simulink library "vehicle_model"  (R2018b)
settings: Solver=ode45  StartTime=0.0  StopTime=10.0  RelTol=1e-3  EnableMultiTasking=on
undefined symbols (not defined in the file): DiscIntNeverNeededParam, par_VEH, select_To_Wks_akt, stepsize, v0
libraries: $bdroot x8, pacejka_trans x6, simulink x4, body_chassis_vert x1
(part 2 of 4)

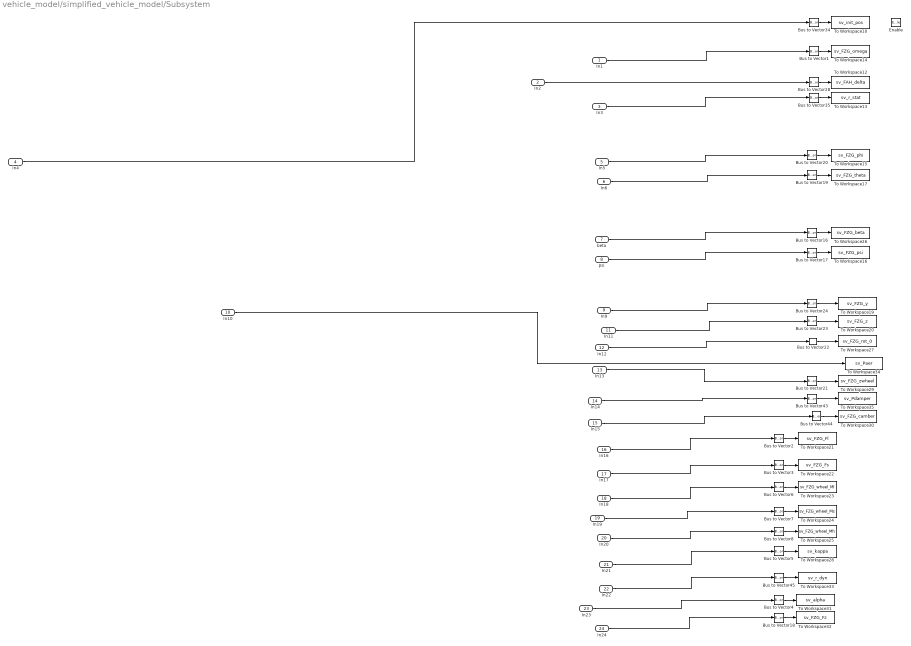
== system vehicle_model/simplified_vehicle_model/Subsystem ==
  In1 : Inport
  In2 : Inport  Port=2
  In3 : Inport  Port=3
  In4 : Inport  Port=4
  In5 : Inport  Port=5
  In6 : Inport  Port=6
  beta : Inport  Port=7
  psi : Inport  Port=8
  In9 : Inport  Port=9
  In10 : Inport  Port=10
  In11 : Inport  Port=11
  In12 : Inport  Port=12
  In13 : Inport  Port=13
  In14 : Inport  Port=14
  In15 : Inport  Port=15
  In16 : Inport  Port=16
  In17 : Inport  Port=17
  In18 : Inport  Port=18
  In19 : Inport  Port=19
  In20 : Inport  Port=20
  In21 : Inport  Port=21
  In22 : Inport  Port=22
  In23 : Inport  Port=23
  In24 : Inport  Port=24
  Enable : EnablePort
  Bus to Vector{1..8,16..24,28,34..35,43..45} (23 alike) : BusToVector
  To Workspace10 : ToWorkspace  VariableName=sv_init_pos  SampleTime=-1
      settings: MaxDataPoints=1  Decimation=savedec  Save2DSignal=2-D array (concatenate along first dimension)
  To Workspace12 : ToWorkspace  VariableName=sv_FAH_delta  SampleTime=-1
      settings: Decimation=savedec  Save2DSignal=2-D array (concatenate along first dimension)
  To Workspace13 : ToWorkspace  VariableName=sv_r_stat  SampleTime=-1
      settings: Decimation=savedec  Save2DSignal=2-D array (concatenate along first dimension)
  To Workspace14 : ToWorkspace  VariableName=sv_FZG_omega  SampleTime=-1
      settings: Decimation=savedec  Save2DSignal=2-D array (concatenate along first dimension)
  To Workspace15 : ToWorkspace  VariableName=sv_FZG_phi  SampleTime=-1
      settings: Decimation=savedec  Save2DSignal=2-D array (concatenate along first dimension)
  To Workspace16 : ToWorkspace  VariableName=sv_FZG_psi  SampleTime=-1
      settings: Decimation=savedec  Save2DSignal=2-D array (concatenate along first dimension)
  To Workspace17 : ToWorkspace  VariableName=sv_FZG_theta  SampleTime=-1
      settings: Decimation=savedec  Save2DSignal=2-D array (concatenate along first dimension)
  To Workspace19 : ToWorkspace  VariableName=sv_FZG_y  SampleTime=-1
      settings: Decimation=savedec  Save2DSignal=2-D array (concatenate along first dimension)
  To Workspace20 : ToWorkspace  VariableName=sv_FZG_z  SampleTime=-1
      settings: Decimation=savedec  Save2DSignal=2-D array (concatenate along first dimension)
  To Workspace21 : ToWorkspace  VariableName=sv_FZG_Fl  SampleTime=-1
      settings: Decimation=savedec  Save2DSignal=2-D array (concatenate along first dimension)
  To Workspace22 : ToWorkspace  VariableName=sv_FZG_Fs  SampleTime=-1
      settings: Decimation=savedec  Save2DSignal=2-D array (concatenate along first dimension)
  To Workspace23 : ToWorkspace  VariableName=sv_FZG_wheel_Ml  SampleTime=-1
      settings: Decimation=savedec  Save2DSignal=2-D array (concatenate along first dimension)
  To Workspace24 : ToWorkspace  VariableName=sv_FZG_wheel_Ms  SampleTime=-1
      settings: Decimation=savedec  Save2DSignal=2-D array (concatenate along first dimension)
  To Workspace25 : ToWorkspace  VariableName=sv_FZG_wheel_Mh  SampleTime=-1
      settings: Decimation=savedec  Save2DSignal=2-D array (concatenate along first dimension)
  To Workspace26 : ToWorkspace  VariableName=sv_FZG_beta  SampleTime=-1
      settings: Decimation=savedec  Save2DSignal=2-D array (concatenate along first dimension)
  To Workspace27 : ToWorkspace  VariableName=sv_FZG_rot_0  SampleTime=-1
      settings: Decimation=savedec  Save2DSignal=2-D array (concatenate along first dimension)
  To Workspace28 : ToWorkspace  VariableName=sv_kappa  SampleTime=-1
      settings: Decimation=savedec  Save2DSignal=2-D array (concatenate along first dimension)
  To Workspace29 : ToWorkspace  VariableName=sv_FZG_zwheel  SampleTime=-1
      settings: Decimation=savedec  Save2DSignal=2-D array (concatenate along first dimension)
  To Workspace30 : ToWorkspace  VariableName=sv_FZG_camber  SampleTime=-1
      settings: Decimation=savedec  Save2DSignal=2-D array (concatenate along first dimension)
  To Workspace31 : ToWorkspace  VariableName=sv_alpha  SampleTime=-1
      settings: Decimation=savedec  Save2DSignal=2-D array (concatenate along first dimension)
  To Workspace32 : ToWorkspace  VariableName=sv_FZG_Fz  SampleTime=-1
      settings: Decimation=savedec  Save2DSignal=2-D array (concatenate along first dimension)
  To Workspace33 : ToWorkspace  VariableName=sv_r_dyn  SampleTime=-1
      settings: Decimation=savedec  Save2DSignal=2-D array (concatenate along first dimension)
  To Workspace34 : ToWorkspace  VariableName=sv_Paer  SampleTime=-1
      settings: Decimation=savedec  Save2DSignal=2-D array (concatenate along first dimension)
  To Workspace35 : ToWorkspace  VariableName=sv_Pdamper  SampleTime=-1
      settings: Decimation=savedec  Save2DSignal=2-D array (concatenate along first dimension)
  wires:
  In2/1 -> Bus to Vector28/1
  Bus to Vector43/1 -> To Workspace35/1
  Bus to Vector35/1 -> To Workspace13/1
  Bus to Vector19/1 -> To Workspace17/1
  Bus to Vector34/1 -> To Workspace10/1
  Bus to Vector8/1 -> To Workspace25/1
  Bus to Vector45/1 -> To Workspace33/1
  Bus to Vector3/1 -> To Workspace22/1
  Bus to Vector20/1 -> To Workspace15/1
  Bus to Vector23/1 -> To Workspace20/1
  Bus to Vector1/1 -> To Workspace14/1
  Bus to Vector21/1 -> To Workspace29/1
  Bus to Vector28/1 -> To Workspace12/1
  Bus to Vector22/1 -> To Workspace27/1
  Bus to Vector2/1 -> To Workspace21/1
  Bus to Vector5/1 -> To Workspace28/1
  In14/1 -> Bus to Vector43/1
  Bus to Vector6/1 -> To Workspace23/1
  Bus to Vector18/1 -> To Workspace32/1
  Bus to Vector17/1 -> To Workspace16/1
  Bus to Vector16/1 -> To Workspace26/1
  Bus to Vector4/1 -> To Workspace31/1
  In23/1 -> Bus to Vector4/1
  In15/1 -> Bus to Vector44/1
  Bus to Vector24/1 -> To Workspace19/1
  Bus to Vector44/1 -> To Workspace30/1
  In10/1 -> To Workspace34/1
  Bus to Vector7/1 -> To Workspace24/1
  In12/1 -> Bus to Vector22/1
  In3/1 -> Bus to Vector35/1
  In19/1 -> Bus to Vector7/1
  In20/1 -> Bus to Vector8/1
  In4/1 -> Bus to Vector34/1
  In1/1 -> Bus to Vector1/1
  In11/1 -> Bus to Vector23/1
  In6/1 -> Bus to Vector19/1
  In9/1 -> Bus to Vector24/1
  In17/1 -> Bus to Vector3/1
  In13/1 -> Bus to Vector21/1
  In16/1 -> Bus to Vector2/1
  In18/1 -> Bus to Vector6/1
  beta/1 -> Bus to Vector16/1
  In5/1 -> Bus to Vector20/1
  psi/1 -> Bus to Vector17/1
  In21/1 -> Bus to Vector5/1
  In22/1 -> Bus to Vector45/1
  In24/1 -> Bus to Vector18/1

== system vehicle_model/simplified_vehicle_model/To workspace activator ==
  road_mu : Inport
  TIR_scale : Inport  Port=2
  TIR_param : Inport  Port=3
  M_brems : Inport  Port=4
  M_antr : Inport  Port=5
  rho_air : Inport  Port=6
  v_wind : Inport  Port=7
  road_orientation : Inport  Port=8
  reset : Inport  Port=9
  FZG_param : Inport  Port=10
  Enable : EnablePort
  Bus to Vector{,26..27,29..33,38} (9 alike) : BusToVector
  To Workspace : ToWorkspace  VariableName=sv_FZG_Parameter  SampleTime=-1
      settings: MaxDataPoints=1  Decimation=savedec  Save2DSignal=2-D array (concatenate along first dimension)
  To Workspace1 : ToWorkspace  VariableName=sv_ENV_v_wind  SampleTime=-1
      settings: Decimation=savedec  Save2DSignal=2-D array (concatenate along first dimension)
  To Workspace11 : ToWorkspace  VariableName=sv_FZG_delta  SampleTime=-1
      settings: Decimation=savedec  Save2DSignal=2-D array (concatenate along first dimension)
  To Workspace2 : ToWorkspace  VariableName=sv_ENV_rho_air  SampleTime=-1
      settings: Decimation=savedec  Save2DSignal=2-D array (concatenate along first dimension)
  To Workspace3 : ToWorkspace  VariableName=sv_reset  SampleTime=-1
      settings: Decimation=savedec  Save2DSignal=2-D array (concatenate along first dimension)
  To Workspace4 : ToWorkspace  VariableName=sv_FZG_M_antr  SampleTime=-1
      settings: Decimation=savedec  Save2DSignal=2-D array (concatenate along first dimension)
  To Workspace5 : ToWorkspace  VariableName=sv_FZG_M_brems  SampleTime=-1
      settings: Decimation=savedec  Save2DSignal=2-D array (concatenate along first dimension)
  To Workspace6 : ToWorkspace  VariableName=sv_TIR_parameter  SampleTime=-1
      settings: MaxDataPoints=1  Decimation=savedec  Save2DSignal=2-D array (concatenate along first dimension)
  To Workspace7 : ToWorkspace  VariableName=sv_TIR_scale  SampleTime=-1
      settings: MaxDataPoints=1  Decimation=savedec  Save2DSignal=2-D array (concatenate along first dimension)
  To Workspace8 : ToWorkspace  VariableName=sv_ENV_road_mu  SampleTime=-1
      settings: Decimation=savedec  Save2DSignal=2-D array (concatenate along first dimension)
  To Workspace9 : ToWorkspace  VariableName=sv_ENV_road_orientation  SampleTime=-1
      settings: Decimation=savedec  Save2DSignal=2-D array (concatenate along first dimension)
  delta : Subsystem
  wires:
  Bus to Vector32/1 -> To Workspace8/1
  Bus to Vector38/1 -> To Workspace5/1
  Bus to Vector30/1 -> To Workspace6/1
  Bus to Vector33/1 -> To Workspace9/1
  Bus to Vector27/1 -> To Workspace1/1
  delta/1(delta) -> Bus to Vector/1
  Bus to Vector/1 -> To Workspace11/1
  Bus to Vector26/1 -> To Workspace/1
  Bus to Vector29/1 -> To Workspace4/1
  Bus to Vector31/1 -> To Workspace7/1
  FZG_param/1 -> Bus to Vector26/1
  road_mu/1 -> Bus to Vector32/1
  rho_air/1 -> To Workspace2/1
  TIR_scale/1 -> Bus to Vector31/1
  v_wind/1 -> Bus to Vector27/1
  M_antr/1 -> Bus to Vector29/1
  TIR_param/1 -> Bus to Vector30/1
  road_orientation/1 -> Bus to Vector33/1
  reset/1 -> To Workspace3/1
  M_brems/1 -> Bus to Vector38/1

== system vehicle_model/simplified_vehicle_model/Transformation ==
  vx : Inport
  vz : Inport  Port=2
  theta : Inport  Port=3
  init_pos : Inport  Port=4
  Add : Sum
  Bus Selector : BusSelector  OutputSignals=init_x0,init_z0
  Constant : Constant  Value=0
  Constant1 : Constant  Value=0
  Discrete-Time Integrator : DiscreteIntegrator  ExternalReset=sampled level  InitialConditionSource=external  SampleTime=-1  ICPrevOutput=DiscIntNeverNeededParam  ICPrevScaledInput=DiscIntNeverNeededParam
  Discrete-Time Integrator2 : DiscreteIntegrator  ExternalReset=sampled level  InitialConditionSource=external  SampleTime=-1  ICPrevOutput=DiscIntNeverNeededParam  ICPrevScaledInput=DiscIntNeverNeededParam
  trafo_matrix : Subsystem
  x0 : Outport
  z0 : Outport  Port=2
  omegax0 : Outport  Port=3
  omegay0 : Outport  Port=4
  omegaz0 : Outport  Port=5
  wires:
  [reset] -> Discrete-Time Integrator2/2, Discrete-Time Integrator/2
  trafo_matrix/1(x0) -> Discrete-Time Integrator/1
  theta/1 -> omegay0/1, trafo_matrix/1(theta)
  Discrete-Time Integrator/1 -> x0/1  "x0"
  Discrete-Time Integrator2/1 -> z0/1  "z0"
  init_pos/1 -> Bus Selector/1
  Bus Selector/1 -> Discrete-Time Integrator/3  "<init_x0>"
  Add/1 -> Discrete-Time Integrator2/3  "<init_z0>"
  vz/1 -> Discrete-Time Integrator2/1
  [zSP] -> Add/2
  Bus Selector/2 -> Add/1  "<init_z0>"
  vx/1 -> trafo_matrix/2(vx)
  Constant/1 -> omegaz0/1
  Constant1/1 -> omegax0/1

== system vehicle_model/simplified_vehicle_model/beta ==
  Bus Creator1 : BusCreator  Inputs=2
  beta : Constant  Value=0
  betap : Constant  Value=0
  Beta : Outport
  wires:
  betap/1 -> Bus Creator1/2  "betap"
  Bus Creator1/1 -> Beta/1
  beta/1 -> Bus Creator1/1  "beta"

== system vehicle_model/simplified_vehicle_model/body_chassis_vert ==
  v_wind : Inport
  rho_air : Inport  Port=2
  Fl : Inport  Port=3
  Fs : Inport  Port=4
  r_stat : Inport  Port=5
  z_wheel : Inport  Port=6
  init_pos : Inport  Port=7
  z_road : Inport  Port=8
  Add : Sum
  Add3 : Sum
  Bus Creator : BusCreator  Inputs=2
  Bus Selector : BusSelector  OutputSignals=Fz_spring_Front,Fz_spring_Rear
  Bus Selector1 : BusSelector  OutputSignals=Fz_damper_Front,Fz_damper_Rear
  Bus Selector2 : BusSelector  OutputSignals=z_vertpp,z_vertp
  Subsystem : Subsystem
  Unit Delay3 : UnitDelay  SampleTime=-1
  horizontal : Subsystem
  kinematics_compliance1 : Subsystem
  pitch : Subsystem
  road_orientation : Subsystem
  suspension : Subsystem
  transformation : Subsystem
  vertical : Subsystem
  a_xz : Outport
  v_xz : Outport  Port=2
  theta : Outport  Port=3
  P_damper : Outport  Port=4
  P_aer : Outport  Port=5
  Fzt : Outport  Port=6
  z_wheel_body : Outport  Port=7
  gamma : Outport  Port=8
  wires:
  vertical/2(F_unsprung_vert) -> Subsystem/3(Fz_unsprung)
  horizontal/3(P_aer) -> P_aer/1
  suspension/4(P_damper) -> P_damper/1
  r_stat/1 -> Unit Delay3/1
  Unit Delay3/1 -> pitch/2(rstat)
  rho_air/1 -> horizontal/2(rho_air)
  init_pos/1 -> vertical/3(init_pos), pitch/5(init_pos)
  v_wind/1 -> horizontal/3(v_wind)
  vertical/1(z_body_vertical) -> suspension/2(z_body_vertical), Bus Selector2/1
  z_wheel/1 -> suspension/3(z_wheel_vertical)
  pitch/2(z_body_pitch) -> suspension/1(z_body_pitch)
  Bus Selector/1 -> Add/1  "<Fz_spring_Front>"
  Bus Selector1/1 -> Add/2  "<Fz_damper_Front>"
  Bus Selector/2 -> Add3/1  "<Fz_spring_Rear>"
  Bus Selector1/2 -> Add3/2  "<Fz_damper_Rear>"
  Add/1 -> Bus Creator/1  "Fz_Front"
  Add3/1 -> Bus Creator/2  "Fz_Rear"
  Bus Selector2/1 -> transformation/3(az)  "<z_vertpp>"
  Bus Selector2/2 -> transformation/4(vz)  "<z_vertp>"
  transformation/2(v_xz) -> v_xz/1
  transformation/1(a_xz) -> a_xz/1
  horizontal/1(ax) -> pitch/1(ax), transformation/1(ax)  "ax"
  horizontal/2(vx) -> transformation/2(vx)  "vx"
  pitch/1(pitch_body) -> theta/1
  Bus Creator/1 -> Subsystem/1(Fz_susp)
  Subsystem/1(Fzt) -> Fzt/1
  pitch/3(F_kin_pitch) -> Subsystem/2(Fz_kinP)
  suspension/2(F_damper) -> vertical/2(Fz_damper), pitch/4(Fz_damper), Bus Selector1/1
  suspension/1(F_spring) -> Bus Selector/1, vertical/1(Fz_spring), pitch/3(Fz_spring)
  suspension/3(z_wheel) -> kinematics_compliance1/1(z), z_wheel_body/1
  z_road/1 -> road_orientation/1(zroad)
  road_orientation/1(theta_road) -> horizontal/4(pitch_road)
  Fs/1 -> kinematics_compliance1/3(Fs)
  Fl/1 -> kinematics_compliance1/2(Fl), horizontal/1(Fl)
  kinematics_compliance1/1(gamma) -> gamma/1

== system vehicle_model/simplified_vehicle_model/phi  ==
  init_pos : Inport
  Bus Creator1 : BusCreator  Inputs=3
  Bus Selector1 : BusSelector  OutputSignals=init_phi
  phip : Constant  Value=0
  phipp : Constant  Value=0
  phi : Outport
  wires:
  phipp/1 -> Bus Creator1/3  "phipp"
  Bus Creator1/1 -> phi/1
  phip/1 -> Bus Creator1/2  "phip"
  init_pos/1 -> Bus Selector1/1  "init_pos"
  Bus Selector1/1 -> Bus Creator1/1  "<init_phi>"

== system vehicle_model/simplified_vehicle_model/psi ==
  Bus Creator1 : BusCreator  Inputs=3
  psi : Constant  Value=0
  psip : Constant  Value=0
  psipp : Constant  Value=0
  Psi : Outport
  wires:
  psipp/1 -> Bus Creator1/3  "psipp"
  Bus Creator1/1 -> Psi/1
  psip/1 -> Bus Creator1/2  "psip"
  psi/1 -> Bus Creator1/1  "psi"

== system vehicle_model/simplified_vehicle_model/wheel ==
  M_antr : Inport
  M_brems : Inport  Port=2
  TIR_parameter : Inport  Port=3
  TIR_scale : Inport  Port=4
  mue_ext : Inport  Port=5
  Init_pos : Inport  Port=6
  v : Inport  Port=7
  Fzt : Inport  Port=8
  gamma : Inport  Port=9
  Bus Creator3 : BusCreator  Inputs=2
  Bus Selector : BusSelector  OutputSignals=vx
  Terminator_11 : Terminator
  Tire_Model : Subsystem
  calc_Fz : Subsystem
  calc_omega : Subsystem
  v0_korr : Subsystem
  wheel_lift : Subsystem
  Fl : Outport
  Fs : Outport  Port=2
  r_stat : Outport  Port=3
  zwheel : Outport  Port=4
  omega_out : Outport  Port=5
  alpha : Outport  Port=6
  kappa : Outport  Port=7
  Mx : Outport  Port=8
  My : Outport  Port=9
  Mz : Outport  Port=10
  r_dyn : Outport  Port=11
  F0 : Outport  Port=12
  wires:
  TIR_scale/1 -> Tire_Model/4(TIR_scale)
  Tire_Model/3(Mx) -> Mx/1
  Tire_Model/4(r_dyn) -> r_dyn/1, v0_korr/2(r_dyn), calc_omega/3(r_dyn)
  Tire_Model/5(My) -> My/1, calc_omega/4(My)
  calc_omega/1(omega) -> Tire_Model/5(omega), v0_korr/3(omega)
  mue_ext/1 -> Tire_Model/7(mue_ext)
  Tire_Model/1(Fl) -> calc_omega/5(Fl), Fl/1
  Tire_Model/6(Mz) -> Mz/1
  Tire_Model/8(kappa) -> kappa/1
  TIR_parameter/1 -> Tire_Model/3(TIR_parameter)
  Tire_Model/9(r_stat) -> r_stat/1, calc_omega/6(r_stat)
  v0_korr/1(omega_out) -> omega_out/1
  Bus Creator3/1 -> calc_Fz/3(zwheel), zwheel/1
  Fzt/1 -> wheel_lift/1(Fz_spring)
  calc_Fz/1(Fztire) -> wheel_lift/2(Fz_tire_wheel), Tire_Model/2(Fz)
  Tire_Model/12(dz) -> calc_Fz/2(dz)
  Tire_Model/11(cz) -> calc_Fz/1(cz)
  wheel_lift/2(zwheel_R) -> Bus Creator3/2  "zwheel_R"
  Init_pos/1 -> wheel_lift/3(init_pos)
  Tire_Model/13(F0) -> F0/1
  wheel_lift/1(zwheel_F) -> Bus Creator3/1  "zwheel_F"
  M_brems/1 -> calc_omega/2(M_brems)
  M_antr/1 -> calc_omega/1(M_antr)
  Tire_Model/10(Aligning_torque_vars) -> Terminator_11/1
  v/1 -> Bus Selector/1
  Bus Selector/1 -> v0_korr/1(vl), Tire_Model/1(v)  "<vx>"
  Tire_Model/2(Fs) -> Fs/1
  gamma/1 -> Tire_Model/6(gamma)
  Tire_Model/7(alpha) -> alpha/1

== system vehicle_model/simplified_vehicle_model/y ==
  y0_init : Inport
  Bus Creator1 : BusCreator  Inputs=3
  Bus Selector2 : BusSelector  OutputSignals=init_y0
  Signal Conversion1 : SignalConversion  OverrideOpt=off
  ay : Constant  Value=0
  vy : Constant  Value=0
  y : Outport
  wires:
  ay/1 -> Bus Creator1/3  "ay"
  Bus Creator1/1 -> y/1
  vy/1 -> Bus Creator1/2  "vy"
  y0_init/1 -> Bus Selector2/1  "y0"
  Bus Selector2/1 -> Signal Conversion1/1  "<init_y0>"
  Signal Conversion1/1 -> Bus Creator1/1  "y0"

== system vehicle_model/vehicle_model/Transformation ==
  vx : Inport
  vy : Inport  Port=2
  vz : Inport  Port=3
  theta : Inport  Port=4
  psi : Inport  Port=5
  phi : Inport  Port=6
  init_pos : Inport  Port=7
  Add : Sum
  Bus Selector : BusSelector  OutputSignals=init_x0,init_y0,init_z0
  Constant : Constant  Value=0
  Demux1 : Demux  Outputs=3
  Demux2 : Demux  Outputs=3
  Discrete-Time Integrator : DiscreteIntegrator  ExternalReset=sampled level  InitialConditionSource=external  SampleTime=-1  ICPrevOutput=DiscIntNeverNeededParam  ICPrevScaledInput=DiscIntNeverNeededParam
  Discrete-Time Integrator1 : DiscreteIntegrator  ExternalReset=sampled level  InitialConditionSource=external  SampleTime=-1  ICPrevOutput=DiscIntNeverNeededParam  ICPrevScaledInput=DiscIntNeverNeededParam
  Discrete-Time Integrator2 : DiscreteIntegrator  ExternalReset=sampled level  InitialConditionSource=external  SampleTime=-1  ICPrevOutput=DiscIntNeverNeededParam  ICPrevScaledInput=DiscIntNeverNeededParam
  Math Function : Math  Operator=transpose  SaturateOnIntegerOverflow=on
  Math Function1 : Math  Operator=transpose  SaturateOnIntegerOverflow=on
  Matrix Concatenate1 : Concatenate  NumInputs=3
  Matrix Concatenate2 : Concatenate  NumInputs=3
  Product : Product  Multiplication=Matrix(*)
  Product1 : Product  Multiplication=Matrix(*)
  Terminator : Terminator
  trafo_matrix : Subsystem
  trafo_matrix1 : Subsystem
  x0 : Outport
  y0 : Outport  Port=2
  z0 : Outport  Port=3
  omegax0 : Outport  Port=4
  omegay0 : Outport  Port=5
  omegaz0 : Outport  Port=6
  wires:
  Product1/1 -> Demux2/1
  trafo_matrix1/1(OTo) -> Math Function1/1
  Math Function1/1 -> Product1/1
  Matrix Concatenate1/1 -> Product1/2
  Product/1 -> Demux1/1
  Demux1/3 -> Terminator/1
  Math Function/1 -> Product/1
  Constant/1 -> Matrix Concatenate2/3
  Matrix Concatenate2/1 -> Product/2
  trafo_matrix/1(OT3) -> Math Function/1
  Bus Selector/3 -> Add/1  "<init_z0>"
  [zSP] -> Add/2
  vz/1 -> Discrete-Time Integrator2/1
  Add/1 -> Discrete-Time Integrator2/3  "<init_z0>"
  Bus Selector/2 -> Discrete-Time Integrator1/3  "<init_y0>"
  Bus Selector/1 -> Discrete-Time Integrator/3  "<init_x0>"
  init_pos/1 -> Bus Selector/1
  Demux2/3 -> omegaz0/1
  Demux2/2 -> omegay0/1
  Demux2/1 -> omegax0/1
  Discrete-Time Integrator2/1 -> z0/1  "z0"
  Discrete-Time Integrator1/1 -> y0/1  "y0"
  Discrete-Time Integrator/1 -> x0/1  "x0"
  vy/1 -> Matrix Concatenate2/2
  vx/1 -> Matrix Concatenate2/1
  phi/1 -> Matrix Concatenate1/3, trafo_matrix/3(phi)
  theta/1 -> trafo_matrix1/2(theta), Matrix Concatenate1/2, trafo_matrix/2(theta)
  psi/1 -> trafo_matrix1/1(psi), Matrix Concatenate1/1, trafo_matrix/1(psi)
  Demux1/2 -> Discrete-Time Integrator1/1
  Demux1/1 -> Discrete-Time Integrator/1
  [reset] -> Discrete-Time Integrator/2, Discrete-Time Integrator1/2, Discrete-Time Integrator2/2

== system vehicle_model/vehicle_model/Transformation1 ==
  psi : Inport
  theta : Inport  Port=2
  phi : Inport  Port=3
  vx : Inport  Port=4
  Bus Creator : BusCreator  Inputs=3
  Bus Selector : BusSelector  OutputSignals=vx,vy,vz
  Bus Selector1 : BusSelector  OutputSignals=psi
  Bus Selector2 : BusSelector  OutputSignals=theta
  Bus Selector3 : BusSelector  OutputSignals=phi
  Demux1 : Demux  Outputs=3
  Math Function : Math  Operator=transpose  SaturateOnIntegerOverflow=on
  Matrix Concatenate2 : Concatenate  NumInputs=3
  Product : Product  Multiplication=Matrix(*)
  trafo_matrix : Subsystem
  x3 : Outport
  wires:
  Product/1 -> Demux1/1
  Math Function/1 -> Product/1
  Matrix Concatenate2/1 -> Product/2
  trafo_matrix/1(OT3) -> Math Function/1
  Bus Selector3/1 -> trafo_matrix/3(phi)  "<phi>"
  Bus Selector2/1 -> trafo_matrix/2(theta)  "<theta>"
  Bus Selector1/1 -> trafo_matrix/1(psi)  "<psi>"
  phi/1 -> Bus Selector3/1
  theta/1 -> Bus Selector2/1
  psi/1 -> Bus Selector1/1
  Demux1/3 -> Bus Creator/3  "vwindz"
  Demux1/2 -> Bus Creator/2  "vwindy"
  Demux1/1 -> Bus Creator/1  "vwindx"
  Bus Selector/3 -> Matrix Concatenate2/3  "<vz>"
  Bus Selector/2 -> Matrix Concatenate2/2  "<vy>"
  Bus Selector/1 -> Matrix Concatenate2/1  "<vx>"
  vx/1 -> Bus Selector/1
  Bus Creator/1 -> x3/1

== system vehicle_model/vehicle_model/calc_init ==
  init_pos : Inport
  Bus Creator : BusCreator  Inputs=10
  Bus Selector : BusSelector  OutputSignals=init_x0,init_y0,init_psi,zroad_RF0,zroad_LF0,zroad_RR0,zroad_LR0
  pitch : Subsystem
  roll : Subsystem
  vertical : Subsystem
  init_pos_complete : Outport
  wires:
  Bus Creator/1 -> init_pos_complete/1
  vertical/1(init_z0) -> Bus Creator/10  "init_z0"
  Bus Selector/7 -> Bus Creator/7  "<zroad_LR0>"
  Bus Selector/6 -> Bus Creator/6  "<zroad_RR0>"
  Bus Selector/5 -> Bus Creator/5  "<zroad_LF0>"
  Bus Selector/4 -> Bus Creator/4  "<zroad_RF0>"
  Bus Selector/3 -> Bus Creator/3  "<init_psi>"
  Bus Selector/2 -> Bus Creator/2  "<init_y0>"
  Bus Selector/1 -> Bus Creator/1  "<init_x0>"
  pitch/1(init_theta) -> vertical/2(theta), Bus Creator/9  "init_theta"
  roll/1(init_phi) -> Bus Creator/8  "init_phi"
  init_pos/1 -> Bus Selector/1, roll/1(init_pos), vertical/1(init_pos), pitch/1(init_pos)

== system vehicle_model/vehicle_model/wheel ==
  M_antr : Inport
  M_brems : Inport  Port=2
  delta : Inport  Port=3
  TIR_parameter : Inport  Port=4
  TIR_scale : Inport  Port=5
  mu_ext : Inport  Port=6
  init_pos : Inport  Port=7
  beta : Inport  Port=8
  psi : Inport  Port=9
  v : Inport  Port=10
  Fzt : Inport  Port=11
  gamma : Inport  Port=12
  z_wheel_body : Inport  Port=13
  Bus Creator3 : BusCreator  Inputs=4
  Terminator_11 : Terminator
  Tire Model : Subsystem
  calc_Fz : Subsystem
  calc_omega : Subsystem
  calc_v : Subsystem
  v0_korr : Subsystem
  wheel_lift : Subsystem
  Fl : Outport
  Fs : Outport  Port=2
  r_stat : Outport  Port=3
  zwheel : Outport  Port=4
  omega_out : Outport  Port=5
  omega : Outport  Port=6
  alpha : Outport  Port=7
  kappa : Outport  Port=8
  Mx : Outport  Port=9
  My : Outport  Port=10
  Mz : Outport  Port=11
  vl : Outport  Port=12
  vs : Outport  Port=13
  r_dyn : Outport  Port=14
  atv : Outport  Port=15
  fric_save : Outport  Port=16
  F0 : Outport  Port=17
  wires:
  Tire Model/13(F0) -> F0/1
  Tire Model/10(aligning_torque_vars) -> atv/1
  Tire Model/12(dz) -> calc_Fz/2(dz)
  M_brems/1 -> calc_omega/2(M_brems)
  Tire Model/4(r_dyn) -> calc_omega/3(r_dyn), v0_korr/2(r_dyn), r_dyn/1
  init_pos/1 -> wheel_lift/3(init_pos)
  Tire Model/9(r_stat) -> calc_omega/8(r_stat), r_stat/1
  Fzt/1 -> wheel_lift/1(Fz_spring)
  calc_Fz/1(Fztire) -> wheel_lift/2(Fz_tire_wheel), calc_omega/6(Fz), Tire Model/2(Fz)
  Tire Model/11(cz) -> calc_Fz/1(cz)
  Bus Creator3/1 -> zwheel/1, calc_Fz/3(zwheel)
  wheel_lift/4(zwheel_LR) -> Bus Creator3/4  "zwheel_LR"
  wheel_lift/3(zwheel_RR) -> Bus Creator3/3  "zwheel_RR"
  wheel_lift/2(zwheel_LF) -> Bus Creator3/2  "zwheel_LF"
  wheel_lift/1(zwheel_RF) -> Bus Creator3/1  "zwheel_RF"
  v0_korr/1(omega_out) -> omega_out/1
  mu_ext/1 -> Tire Model/8(mue_ext)
  Tire Model/1(Fl) -> calc_omega/5(Fl), Fl/1
  Tire Model/5(My) -> calc_omega/4(My), My/1
  calc_omega/1(omega) -> Tire Model/7(omega), omega/1, v0_korr/3(omega)
  calc_v/2(vl) -> Tire Model/1(vl), v0_korr/1(vl), vl/1
  calc_v/1(vs) -> vs/1, Tire Model/6(vs)
  calc_omega/2(omegap) -> Terminator_11/1
  delta/1 -> calc_omega/9(delta), calc_v/1(delta)
  psi/1 -> calc_v/3(psi)
  beta/1 -> calc_v/2(beta)
  M_antr/1 -> calc_omega/1(M_antr)
  Tire Model/2(Fs) -> calc_omega/7(Fs), Fs/1
  Tire Model/3(Mx) -> calc_omega/12(M_x), Mx/1
  gamma/1 -> calc_omega/10(camber), Tire Model/3(gamma)
  TIR_parameter/1 -> Tire Model/4(TIR_parameter)
  TIR_scale/1 -> Tire Model/5(TIR_scale)
  Tire Model/6(Mz) -> calc_omega/13(M_z), Mz/1
  Tire Model/7(alpha) -> alpha/1
  Tire Model/8(kappa) -> kappa/1
  v/1 -> calc_v/4(v)
  calc_omega/3(fric_save) -> fric_save/1
  z_wheel_body/1 -> calc_omega/11(z_wheel_body)

== system vehicle_model/vehicle_model/Überlagerung ==
  spuraenderungen : Inport
  lenkwinkel : Inport  Port=2
  Bus Creator : BusCreator  Inputs=4
  Bus Selector1 : BusSelector  OutputSignals=d_delta_RF,d_delta_LF,d_delta_RR,d_delta_LR
  Bus Selector9 : BusSelector  OutputSignals=delta_RF,delta_LF,delta_RR,delta_LR
  Sum{,1..3} (4 alike) : Sum
  Unit Delay{1..4} (4 alike) : UnitDelay  SampleTime=-1
  ges_lenkwinkel : Outport
  wires:
  Sum/1 -> Bus Creator/2  "delta_LF"
  Bus Creator/1 -> ges_lenkwinkel/1
  Unit Delay4/1 -> Sum3/1
  Unit Delay3/1 -> Sum2/1
  Unit Delay1/1 -> Sum1/1
  Unit Delay2/1 -> Sum/1
  Sum3/1 -> Bus Creator/3  "delta_RR"
  Sum2/1 -> Bus Creator/4  "delta_LR"
  Sum1/1 -> Bus Creator/1  "delta_RF"
  Bus Selector9/4 -> Sum2/2  "<delta_LR>"
  Bus Selector9/3 -> Sum3/2  "<delta_RR>"
  Bus Selector9/2 -> Sum/2  "<delta_LF>"
  Bus Selector9/1 -> Sum1/2  "<delta_RF>"
  Bus Selector1/3 -> Unit Delay4/1  "<d_delta_RR>"
  Bus Selector1/4 -> Unit Delay3/1  "<d_delta_LR>"
  Bus Selector1/1 -> Unit Delay1/1  "<d_delta_RF>"
  Bus Selector1/2 -> Unit Delay2/1  "<d_delta_LF>"
  spuraenderungen/1 -> Bus Selector1/1
  lenkwinkel/1 -> Bus Selector9/1

== system vehicle_model/simplified_vehicle_model/To workspace activator/delta ==
  Bus Creator : BusCreator  Inputs=4
  delta_LF : Constant  Value=0
  delta_LR : Constant  Value=0
  delta_RF : Constant  Value=0
  delta_RR : Constant  Value=0
  delta : Outport
  wires:
  Bus Creator/1 -> delta/1
  delta_LF/1 -> Bus Creator/2  "delta_LF"
  delta_RR/1 -> Bus Creator/3  "delta_RR"
  delta_RF/1 -> Bus Creator/1  "delta_RF"
  delta_LR/1 -> Bus Creator/4  "delta_LR"

== system vehicle_model/simplified_vehicle_model/Transformation/trafo_matrix ==
  theta : Inport
  vx : Inport  Port=2
  Product : Product
  Trigonometric Function2 : Trigonometry  Operator=cos
  x0 : Outport
  wires:
  Trigonometric Function2/1 -> Product/1
  theta/1 -> Trigonometric Function2/1
  Product/1 -> x0/1
  vx/1 -> Product/2

== system vehicle_model/simplified_vehicle_model/body_chassis_vert/Subsystem ==
  Fz_susp : Inport
  Fz_kinP : Inport  Port=2
  Fz_unsprung : Inport  Port=3
  Bus Creator : BusCreator  Inputs=2
  Bus Selector : BusSelector  OutputSignals=Fz_Front,Fz_Rear
  Bus Selector2 : BusSelector  OutputSignals=F_kinP_F,F_kinP_R
  Bus Selector3 : BusSelector  OutputSignals=F_us_Front,F_us_Rear
  Front : Sum  Inputs=+++
  Rear : Sum  Inputs=+++
  Fzt : Outport
  wires:
  Bus Selector3/2 -> Rear/3  "<F_us_Rear>"
  Bus Selector3/1 -> Front/3  "<F_us_Front>"
  Fz_unsprung/1 -> Bus Selector3/1
  Fz_susp/1 -> Bus Selector/1
  Fz_kinP/1 -> Bus Selector2/1
  Bus Selector/1 -> Front/1  "<Fz_Front>"
  Bus Selector/2 -> Rear/1  "<Fz_Rear>"
  Bus Selector2/1 -> Front/2  "<F_kinP_F>"
  Front/1 -> Bus Creator/1  "Fz_Front"
  Rear/1 -> Bus Creator/2  "Fz_Rear"
  Bus Creator/1 -> Fzt/1
  Bus Selector2/2 -> Rear/2  "<F_kinP_R>"

== system vehicle_model/simplified_vehicle_model/body_chassis_vert/horizontal ==
  Fl : Inport
  rho_air : Inport  Port=2
  v_wind : Inport  Port=3
  pitch_road : Inport  Port=4
  Discrete-Time Integrator2 : DiscreteIntegrator  ExternalReset=sampled level  InitialCondition=v0  SampleTime=-1  ICPrevOutput=DiscIntNeverNeededParam  ICPrevScaledInput=DiscIntNeverNeededParam
  "P_aer " : Subsystem
  Product : Product
  Unit Delay3 : UnitDelay  SampleTime=-1
  acc : Subsystem
  aerodynamics : Subsystem
  ax : Outport
  vx : Outport  Port=2
  P_aer : Outport  Port=3
  wires:
  Product/1 -> "P_aer "/1(P_aer_x)
  Unit Delay3/1 -> acc/1(Fl)
  acc/1(a) -> ax/1, Discrete-Time Integrator2/1
  Discrete-Time Integrator2/1 -> vx/1, Product/1, aerodynamics/2(v)  "v"
  aerodynamics/1(F_aer) -> acc/3(F_aer), Product/2
  Fl/1 -> Unit Delay3/1  "Fl"
  rho_air/1 -> aerodynamics/1(rho_air)
  [reset] -> Discrete-Time Integrator2/2
  v_wind/1 -> aerodynamics/3(v_wind)
  pitch_road/1 -> acc/2(pitch)
  "P_aer "/1(P_aer) -> P_aer/1

== system vehicle_model/simplified_vehicle_model/body_chassis_vert/kinematics_compliance1 ==
  note: Spur im FZG-Modell positiv,
      | wenn das Rad nach links gedreht ist
      | (positive z-Achsen-Rotation)
  note: Sturz für FZG-Modell
      | positive wenn Rad oben
      | nach rechts wandert
  note: Kompensation über Lenkwinkel
      | (Rollwinkel wirkt sich bei 90° Lenkwinkel nicht auf den Sturz aus)
  note: Fs positiv wenn
      | Kraft nach links zeigt
  note: Fs für Kennlinie positiv,
      | wenn Kraft nach innen gerichtet
      |
      | Sturz für Kennlinie positiv,
      | wenn das Rad oben nach
      | außen wandert
  note: Spur in der Kennlinie positiv,
      | wenn in Vorspurlage, d.h. nach
      | Fahrzeuginnen gerichtet
  z : Inport
  Fl : Inport  Port=2
  Fs : Inport  Port=3
  Add{4,6,8,10} (4 alike) : Sum
  Bus Creator : BusCreator  Inputs=2
  Bus Selector : BusSelector  OutputSignals=z_wheel_Front,z_wheel_Rear
  Bus Selector3 : BusSelector  OutputSignals=Fs_F,Fs_R
  Bus Selector4 : BusSelector  OutputSignals=Fl_F,Fl_R
  Constant2 : Constant  Value=par_VEH.sw_kinematics
  Constant3 : Constant  Value=par_VEH.sw_compliance
  D2R{3,5,7,14..16} (6 alike) : Gain  Gain=pi/180
  Product{6,8,10,12} (4 alike) : Product  RndMeth=Zero
  Sturz_F1 : Polyval  Coefs=par_VEH.kin_camb_f
  Sturz_R1 : Polyval  Coefs=par_VEH.kin_camb_r
  Unit Delay : UnitDelay  SampleTime=-1
  Unit Delay1 : UnitDelay  SampleTime=-1
  x_camb_f1 : Polyval  Coefs=par_VEH.elkin_x_camb_f
  x_camp_r1 : Polyval  Coefs=par_VEH.elkin_x_camb_r
  y_camb_f1 : Polyval  Coefs=par_VEH.elkin_y_camb_f
  y_camb_r1 : Polyval  Coefs=par_VEH.elkin_y_camb_r
  gamma : Outport
  wires:
  Product8/1 -> Add10/2  "compliance_camber_R"
  Product6/1 -> Add8/2  "compliance_camber_F"
  Add8/1 -> Bus Creator/1  "gamma_F"
  Product12/1 -> Add10/1
  Product10/1 -> Add8/1
  Constant2/1 -> Product12/2, Product10/2
  D2R7/1 -> Product10/1  "Sturz_F"
  Add10/1 -> Bus Creator/2  "gamma_R"
  Constant3/1 -> Product6/1, Product8/1
  D2R3/1 -> Product12/1  "Sturz_R"
  z/1 -> Bus Selector/1
  Sturz_R1/1 -> D2R3/1
  Bus Creator/1 -> gamma/1
  D2R5/1 -> Add6/2  "camber_R_lon"
  D2R16/1 -> Add4/2  "camber_F_lon"
  D2R15/1 -> Add6/1  "camber_R_lat"
  D2R14/1 -> Add4/1  "camber_F_lat"
  Bus Selector4/2 -> x_camp_r1/1  "<Fl_R>"
  Bus Selector4/1 -> x_camb_f1/1  "<Fl_F>"
  Bus Selector3/2 -> y_camb_r1/1  "<Fs_R>"
  Bus Selector3/1 -> y_camb_f1/1  "<Fs_F>"
  Fl/1 -> Unit Delay1/1
  Fs/1 -> Unit Delay/1
  Unit Delay/1 -> Bus Selector3/1
  Unit Delay1/1 -> Bus Selector4/1
  Add4/1 -> Product6/2  "compliance_camber_F"
  Add6/1 -> Product8/2  "compliance_camber_R"
  x_camp_r1/1 -> D2R5/1
  x_camb_f1/1 -> D2R16/1
  y_camb_r1/1 -> D2R15/1
  y_camb_f1/1 -> D2R14/1
  Bus Selector/1 -> Sturz_F1/1  "<z_wheel_Front>"
  Sturz_F1/1 -> D2R7/1
  Bus Selector/2 -> Sturz_R1/1  "<z_wheel_Rear>"

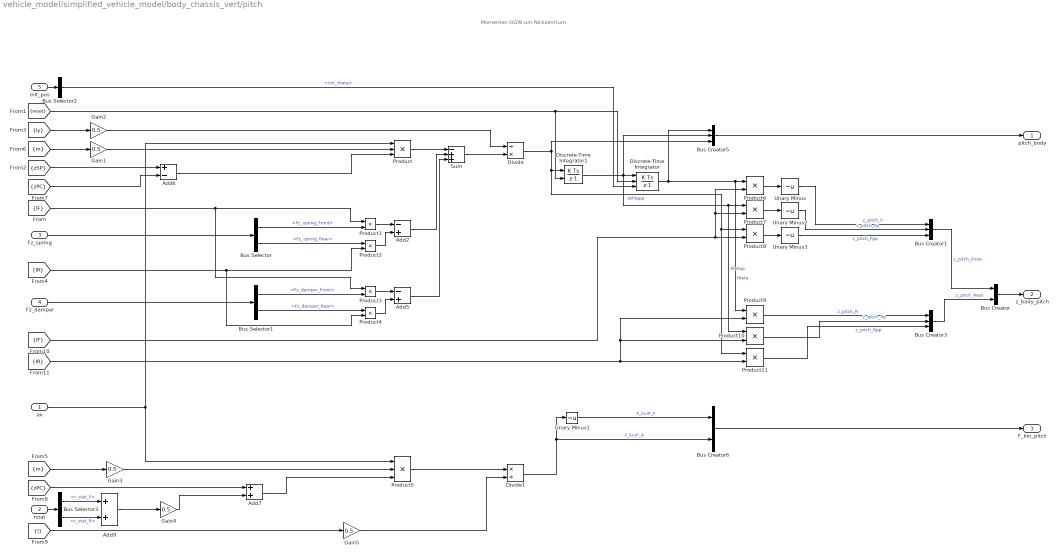
== system vehicle_model/simplified_vehicle_model/body_chassis_vert/pitch ==
  note: Momenten-GGW um Nickzentrum
  ax : Inport
  rstat : Inport  Port=2
  Fz_spring : Inport  Port=3
  Fz_damper : Inport  Port=4
  init_pos : Inport  Port=5
  Add2 : Sum  Inputs=-+
  Add5 : Sum  Inputs=-+
  Add6 : Sum  Inputs=+-
  Add7 : Sum
  Add9 : Sum
  Bus Creator : BusCreator  Inputs=2
  Bus Creator1 : BusCreator  Inputs=3
  Bus Creator3 : BusCreator  Inputs=3
  Bus Creator5 : BusCreator  Inputs=3
  Bus Creator6 : BusCreator  Inputs=2
  Bus Selector : BusSelector  OutputSignals=Fz_spring_Front,Fz_spring_Rear
  Bus Selector1 : BusSelector  OutputSignals=Fz_damper_Front,Fz_damper_Rear
  Bus Selector2 : BusSelector  OutputSignals=init_theta
  Bus Selector3 : BusSelector  OutputSignals=r_stat_F,r_stat_R
  Discrete-Time Integrator : DiscreteIntegrator  ExternalReset=sampled level  InitialConditionSource=external  SampleTime=stepsize  ICPrevOutput=DiscIntNeverNeededParam  ICPrevScaledInput=DiscIntNeverNeededParam
  Discrete-Time Integrator1 : DiscreteIntegrator  ExternalReset=sampled level  SampleTime=stepsize  ICPrevOutput=DiscIntNeverNeededParam  ICPrevScaledInput=DiscIntNeverNeededParam
  Divide : Product  Inputs=/*
  Divide1 : Product  Inputs=*/
  Gain{1..5} (5 alike) : Gain  Gain=0.5
  Product : Product  Inputs=3  RndMeth=Zero
  Product{1..4,6..11} (10 alike) : Product  RndMeth=Zero
  Product5 : Product  Inputs=3  RndMeth=Zero
  Sum : Sum  Inputs=-++
  Unary Minus{,1..3} (4 alike) : UnaryMinus
  pitch_body : Outport
  z_body_pitch : Outport  Port=2
  F_kin_pitch : Outport  Port=3
  wires:
  Product7/1 -> Unary Minus2/1
  Product6/1 -> Unary Minus/1
  Product8/1 -> Unary Minus3/1
  Product11/1 -> Bus Creator3/3  "z_pitch_Rpp"
  Product10/1 -> Bus Creator3/2  "z_pitch_Rp"
  Product9/1 -> Bus Creator3/1  "z_pitch_R"
  [lR] -> Product11/2, Product10/2, Product9/2
  [lF] -> Product6/2, Product7/2, Product8/2
  [lF] -> Product3/1, Product1/1
  [lR] -> Product4/2, Product2/2
  [m] -> Gain3/1
  Bus Creator6/1 -> F_kin_pitch/1
  Product5/1 -> Divide1/1
  [l] -> Gain5/1
  Add7/1 -> Product5/3
  Add2/1 -> Sum/2
  Add5/1 -> Sum/3
  Product/1 -> Sum/1
  Add6/1 -> Product/3
  Unary Minus3/1 -> Bus Creator1/3  "z_pitch_Fpp"
  Unary Minus/1 -> Bus Creator1/1  "z_pitch_F"
  Product4/1 -> Add5/2
  Product3/1 -> Add5/1
  Bus Selector1/2 -> Product4/1  "<Fz_damper_Rear>"
  Bus Selector1/1 -> Product3/2  "<Fz_damper_Front>"
  Product2/1 -> Add2/2
  Product1/1 -> Add2/1
  Fz_damper/1 -> Bus Selector1/1
  Bus Selector/2 -> Product2/1  "<Fz_spring_Rear>"
  Bus Selector/1 -> Product1/2  "<Fz_spring_Front>"
  Fz_spring/1 -> Bus Selector/1
  Discrete-Time Integrator1/1 -> Bus Creator5/2, Product7/1, Product10/1, Discrete-Time Integrator/1  "thetap"
  Divide/1 -> Bus Creator5/3, Discrete-Time Integrator1/1, Product11/1, Product8/1  "tehtapp"
  [Iy] -> Gain2/1
  Sum/1 -> Divide/2
  [m] -> Gain1/1
  Bus Creator5/1 -> pitch_body/1
  Discrete-Time Integrator/1 -> Product6/1, Product9/1, Bus Creator5/1  "theta"
  Unary Minus2/1 -> Bus Creator1/2  "z_pitch_Fp"
  Bus Creator3/1 -> Bus Creator/2  "z_pitch_Rear"
  Bus Creator1/1 -> Bus Creator/1  "z_pitch_Front"
  Bus Creator/1 -> z_body_pitch/1
  init_pos/1 -> Bus Selector2/1
  Bus Selector2/1 -> Discrete-Time Integrator/3  "<init_theta>"
  [reset] -> Discrete-Time Integrator1/2, Discrete-Time Integrator/2
  [zSP] -> Add6/1
  [zPC] -> Add6/2
  [zPC] -> Add7/1
  Add9/1 -> Gain4/1
  Bus Selector3/1 -> Add9/1  "<r_stat_F>"
  Bus Selector3/2 -> Add9/2  "<r_stat_R>"
  rstat/1 -> Bus Selector3/1
  Gain4/1 -> Add7/2
  Divide1/1 -> Unary Minus1/1, Bus Creator6/2  "F_kinP_R"
  ax/1 -> Product5/1, Product/1
  Unary Minus1/1 -> Bus Creator6/1  "F_kinP_F"
  Gain1/1 -> Product/2
  Gain2/1 -> Divide/1
  Gain3/1 -> Product5/2
  Gain5/1 -> Divide1/2

== system vehicle_model/simplified_vehicle_model/body_chassis_vert/road_orientation ==
  zroad : Inport
  Bus Selector1 : BusSelector  OutputSignals=zroad_RF,zroad_LF,zroad_RR,zroad_LR
  Divide8 : Product  Inputs=*/
  Gain3 : Gain  Gain=0.5
  Gain4 : Gain  Gain=0.5
  Subtract18 : Sum
  Subtract19 : Sum
  Subtract20 : Sum  Inputs=+-
  Trigonometric Function : Trigonometry  Operator=asin
  theta_road : Outport
  wires:
  zroad/1 -> Bus Selector1/1
  Bus Selector1/3 -> Subtract19/1  "<zroad_RR>"
  Bus Selector1/2 -> Subtract18/2  "<zroad_LF>"
  Bus Selector1/4 -> Subtract19/2  "<zroad_LR>"
  Trigonometric Function/1 -> theta_road/1
  Bus Selector1/1 -> Subtract18/1  "<zroad_RF>"
  Subtract18/1 -> Gain3/1
  Subtract19/1 -> Gain4/1
  Gain3/1 -> Subtract20/1
  Gain4/1 -> Subtract20/2
  Subtract20/1 -> Divide8/1
  [l] -> Divide8/2
  Divide8/1 -> Trigonometric Function/1

== system vehicle_model/simplified_vehicle_model/body_chassis_vert/suspension ==
  z_body_pitch : Inport
  z_body_vertical : Inport  Port=2
  z_wheel_vertical : Inport  Port=3
  damper : Subsystem
  spring : Subsystem
  F_spring : Outport
  F_damper : Outport  Port=2
  z_wheel : Outport  Port=3
  P_damper : Outport  Port=4
  wires:
  damper/2(P_damper) -> P_damper/1
  damper/1(F_damper) -> F_damper/1
  z_body_pitch/1 -> damper/1(z_pitch), spring/1(z_pitch)
  z_body_vertical/1 -> damper/2(z_body_vert), spring/2(z_vert)
  z_wheel_vertical/1 -> damper/3(z_wheel_vert), spring/3(z_wheel_vert)
  spring/2(z_wheel) -> z_wheel/1
  spring/1(Fz_spring) -> F_spring/1

== system vehicle_model/simplified_vehicle_model/body_chassis_vert/transformation ==
  ax : Inport
  vx : Inport  Port=2
  az : Inport  Port=3
  vz : Inport  Port=4
  Bus Creator1 : BusCreator  Inputs=2
  Bus Creator2 : BusCreator  Inputs=2
  a_xz : Outport
  v_xz : Outport  Port=2
  wires:
  ax/1 -> Bus Creator1/1  "ax"
  Bus Creator1/1 -> a_xz/1
  az/1 -> Bus Creator1/2  "az"
  vx/1 -> Bus Creator2/1  "vx"
  Bus Creator2/1 -> v_xz/1
  vz/1 -> Bus Creator2/2  "vz"

== system vehicle_model/simplified_vehicle_model/body_chassis_vert/vertical ==
  Fz_spring : Inport
  Fz_damper : Inport  Port=2
  init_pos : Inport  Port=3
  Add : Sum  Inputs=+--
  Add1 : Sum  Inputs=++++-
  Bus Creator : BusCreator  Inputs=3
  Bus Creator1 : BusCreator  Inputs=2
  Bus Selector : BusSelector  OutputSignals=Fz_spring_Front,Fz_spring_Rear
  Bus Selector1 : BusSelector  OutputSignals=Fz_damper_Front,Fz_damper_Rear
  Bus Selector2 : BusSelector  OutputSignals=init_z0
  Discrete-Time Integrator : DiscreteIntegrator  ExternalReset=sampled level  SampleTime=-1  ICPrevOutput=DiscIntNeverNeededParam  ICPrevScaledInput=DiscIntNeverNeededParam
  Discrete-Time Integrator1 : DiscreteIntegrator  ExternalReset=sampled level  InitialConditionSource=external  SampleTime=-1  ICPrevOutput=DiscIntNeverNeededParam  ICPrevScaledInput=DiscIntNeverNeededParam
  Divide : Product  Inputs=*/
  Gain1 : Gain  Gain=0.5
  Gain2 : Gain  Gain=0.5
  Gain3 : Gain  Gain=0.5
  Product : Product  RndMeth=Zero
  Product1 : Product  RndMeth=Zero
  Product3 : Product  RndMeth=Zero
  Signal Conversion1 : SignalConversion  OverrideOpt=off
  Signal Conversion2 : SignalConversion  OverrideOpt=off
  z_body_vertical : Outport
  F_unsprung_vert : Outport  Port=2
  wires:
  Gain3/1 -> Signal Conversion1/1
  Signal Conversion2/1 -> Bus Creator1/1  "F_us_Front"
  Gain2/1 -> Signal Conversion2/1
  Signal Conversion1/1 -> Bus Creator1/2  "F_us_Rear"
  Bus Creator1/1 -> F_unsprung_vert/1
  Product3/1 -> Gain3/1
  Product1/1 -> Gain2/1
  [m_usR] -> Product3/2
  [g] -> Product1/2, Product3/1
  [m_usF] -> Product1/1
  [m] -> Add/1
  [m_usF] -> Add/2
  [m_usR] -> Add/3
  Add/1 -> Gain1/1
  Discrete-Time Integrator/1 -> Discrete-Time Integrator1/1, Bus Creator/2  "z_vertp"
  Divide/1 -> Discrete-Time Integrator/1, Bus Creator/3  "z_vertpp"
  Bus Creator/1 -> z_body_vertical/1
  Discrete-Time Integrator1/1 -> Bus Creator/1  "z_vert"
  Fz_spring/1 -> Bus Selector/1
  Fz_damper/1 -> Bus Selector1/1
  Bus Selector/1 -> Add1/1  "<Fz_spring_Front>"
  Bus Selector/2 -> Add1/2  "<Fz_spring_Rear>"
  Bus Selector1/1 -> Add1/3  "<Fz_damper_Front>"
  Bus Selector1/2 -> Add1/4  "<Fz_damper_Rear>"
  [reset] -> Discrete-Time Integrator/2, Discrete-Time Integrator1/2
  Bus Selector2/1 -> Discrete-Time Integrator1/3  "<init_z0>"
  init_pos/1 -> Bus Selector2/1
  Product/1 -> Add1/5
  Add1/1 -> Divide/1
  [g] -> Product/1
  Gain1/1 -> Product/2, Divide/2

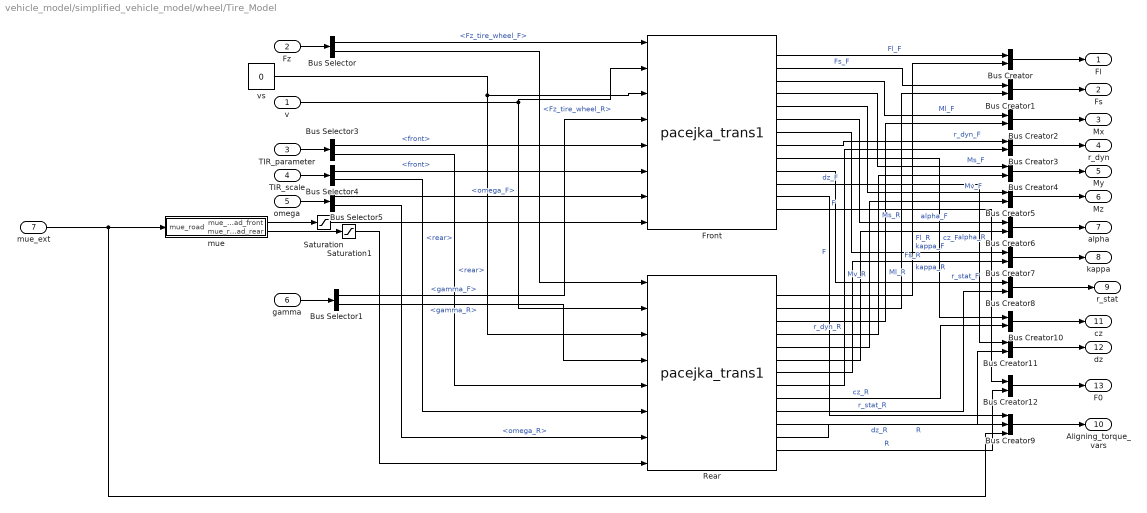
== system vehicle_model/simplified_vehicle_model/wheel/Tire_Model ==
  v : Inport
  Fz : Inport  Port=2
  TIR_parameter : Inport  Port=3
  TIR_scale : Inport  Port=4
  omega : Inport  Port=5
  gamma : Inport  Port=6
  mue_ext : Inport  Port=7
  Bus Creator{,1..8,10..12} (12 alike) : BusCreator  Inputs=2
  Bus Creator9 : BusCreator  Inputs=3
  Bus Selector : BusSelector  OutputSignals=Fz_tire_wheel_F,Fz_tire_wheel_R
  Bus Selector1 : BusSelector  OutputSignals=gamma_F,gamma_R
  Bus Selector3 : BusSelector  OutputSignals=front,rear
  Bus Selector4 : BusSelector  OutputSignals=front,rear
  Bus Selector5 : BusSelector  OutputSignals=omega_F,omega_R
  Front : pacejka_trans/pacejka_trans1  mounted_side_input=right
  Rear : pacejka_trans/pacejka_trans1  mounted_side_input=right
  Saturation : Saturate  UpperLimit=2  LowerLimit=0.05
  Saturation1 : Saturate  UpperLimit=2  LowerLimit=0.05
  mue : Subsystem
  vs : Constant  Value=0
  Fl : Outport
  Fs : Outport  Port=2
  Mx : Outport  Port=3
  r_dyn : Outport  Port=4
  My : Outport  Port=5
  Mz : Outport  Port=6
  alpha : Outport  Port=7
  kappa : Outport  Port=8
  r_stat : Outport  Port=9
  Aligning_torque_vars : Outport  Port=10
  cz : Outport  Port=11
  dz : Outport  Port=12
  F0 : Outport  Port=13
  wires:
  Front/10 -> Bus Creator8/1  "r_stat_F"
  Rear/3 -> Bus Creator2/2  "Ml_R"
  Front/8 -> Bus Creator3/1  "r_dyn_F"
  Rear/10 -> Bus Creator8/2  "r_stat_R"
  Front/5 -> Bus Creator5/1  "Mv_F"
  Bus Selector/2 -> Rear/1  "<Fz_tire_wheel_R>"
  Saturation1/1 -> Rear/8
  Bus Selector/1 -> Front/1  "<Fz_tire_wheel_F>"
  TIR_parameter/1 -> Bus Selector3/1
  Bus Selector4/1 -> Front/6  "<front>"
  Front/1 -> Bus Creator/1  "Fl_F"
  Saturation/1 -> Front/8
  Fz/1 -> Bus Selector/1
  Bus Selector4/2 -> Rear/6  "<rear>"
  Bus Selector1/1 -> Front/4  "<gamma_F>"
  Bus Selector3/1 -> Front/5  "<front>"
  omega/1 -> Bus Selector5/1
  TIR_scale/1 -> Bus Selector4/1
  Bus Selector3/2 -> Rear/5  "<rear>"
  Bus Selector5/1 -> Front/7  "<omega_F>"
  Bus Selector5/2 -> Rear/7  "<omega_R>"
  mue_ext/1 -> Bus Creator9/3, mue/1("mue_road ")
  Bus Creator1/1 -> Fs/1
  Bus Creator2/1 -> Mx/1
  Bus Creator5/1 -> Mz/1
  Rear/2 -> Bus Creator1/2  "Fs_R"
  Bus Creator12/1 -> F0/1
  Bus Creator9/1 -> Aligning_torque_vars/1
  Bus Creator/1 -> Fl/1
  Front/2 -> Bus Creator1/1  "Fs_F"
  Bus Creator6/1 -> alpha/1
  Bus Creator3/1 -> r_dyn/1
  Bus Creator7/1 -> kappa/1
  Bus Creator4/1 -> My/1
  Rear/1 -> Bus Creator/2  "Fl_R"
  Bus Creator11/1 -> dz/1
  Bus Creator10/1 -> cz/1
  Bus Creator8/1 -> r_stat/1
  Rear/9 -> Bus Creator10/2  "cz_R"
  Front/3 -> Bus Creator2/1  "Ml_F"
  Front/7 -> Bus Creator7/1  "kappa_F"
  Rear/8 -> Bus Creator3/2  "r_dyn_R"
  Rear/11 -> Bus Creator11/2  "dz_R"
  Front/11 -> Bus Creator11/1  "dz_F"
  Rear/12 -> Bus Creator9/2  "R"
  Front/13 -> Bus Creator12/1  "F"
  Front/6 -> Bus Creator6/1  "alpha_F"
  Front/12 -> Bus Creator9/1  "F"
  Front/4 -> Bus Creator4/1  "Ms_F"
  Rear/5 -> Bus Creator5/2  "Mv_R"
  Rear/6 -> Bus Creator6/2  "alpha_R"
  Rear/4 -> Bus Creator4/2  "Ms_R"
  Rear/13 -> Bus Creator12/2  "R"
  Front/9 -> Bus Creator10/1  "cz_F"
  Rear/7 -> Bus Creator7/2  "kappa_R"
  vs/1 -> Front/3, Rear/3
  v/1 -> Rear/2, Front/2
  mue/1(mue_road_front) -> Saturation/1
  mue/2(mue_road_rear) -> Saturation1/1
  gamma/1 -> Bus Selector1/1
  Bus Selector1/2 -> Rear/4  "<gamma_R>"

== system vehicle_model/simplified_vehicle_model/wheel/calc_Fz ==
  cz : Inport
  dz : Inport  Port=2
  zwheel : Inport  Port=3
  Bus Creator1 : BusCreator  Inputs=2
  Bus Selector1 : BusSelector  OutputSignals=cz_F,cz_R
  Bus Selector3 : BusSelector  OutputSignals=zwheel_F.zwheel,zwheel_R.zwheel
  Bus Selector4 : BusSelector  OutputSignals=zwheel_F.zwheelp,zwheel_R.zwheelp
  Bus Selector5 : BusSelector  OutputSignals=dz_F,dz_R
  Gain : Gain  Gain=-1
  Gain1 : Gain
  Gain2 : Gain  Gain=-1
  Gain5 : Gain
  Product{,1,4..5} (4 alike) : Product  RndMeth=Zero
  Sum4 : Sum  Inputs=|+-
  Sum5 : Sum  Inputs=|+-
  Fztire : Outport
  wires:
  Gain1/1 -> Product5/2
  Gain5/1 -> Product4/2
  Bus Selector5/2 -> Gain1/1  "<dz_R>"
  Bus Selector5/1 -> Gain5/1  "<dz_F>"
  dz/1 -> Bus Selector5/1
  Product5/1 -> Sum5/2
  Product4/1 -> Sum4/2
  Bus Selector4/1 -> Product4/1  "<zwheelp>"
  Bus Selector4/2 -> Product5/1  "<zwheelp>"
  Sum5/1 -> Bus Creator1/2  "Fz_tire_wheel_R"
  Sum4/1 -> Bus Creator1/1  "Fz_tire_wheel_F"
  Product/1 -> Sum4/1  "Fz_tire_wheel_F"
  Product1/1 -> Sum5/1  "Fz_tire_wheel_R"
  Bus Selector3/2 -> Gain2/1  "<zwheel>"
  Bus Selector3/1 -> Gain/1  "<zwheel>"
  zwheel/1 -> Bus Selector4/1, Bus Selector3/1
  Bus Creator1/1 -> Fztire/1
  Bus Selector1/2 -> Product1/1  "<cz_R>"
  cz/1 -> Bus Selector1/1
  Bus Selector1/1 -> Product/1  "<cz_F>"
  Gain/1 -> Product/2
  Gain2/1 -> Product1/2

== system vehicle_model/simplified_vehicle_model/wheel/calc_omega ==
  M_antr : Inport
  M_brems : Inport  Port=2
  r_dyn : Inport  Port=3
  My : Inport  Port=4
  Fl : Inport  Port=5
  r_stat : Inport  Port=6
  Add : Sum  Inputs=++--
  Add1 : Sum  Inputs=++--
  Add{2..7} (6 alike) : Sum
  Bus Creator : BusCreator  Inputs=2
  Bus Selector2 : BusSelector  OutputSignals=r_stat_F,r_stat_R
  Bus Selector3 : BusSelector  OutputSignals=Ms_F,Ms_R
  Bus Selector4 : BusSelector  OutputSignals=Fl_F,Fl_R
  Bus Selector6 : BusSelector  OutputSignals=r_dyn_F,r_dyn_R
  Bus Selector7 : BusSelector  OutputSignals=M_antr_RF,M_antr_LF,M_antr_RR,M_antr_LR
  Bus Selector8 : BusSelector  OutputSignals=M_brems_RF,M_brems_LF,M_brems_RR,M_brems_LR
  Constant : Constant  Value=v0
  Discrete-Time Integrator1 : DiscreteIntegrator  ExternalReset=sampled level  InitialConditionSource=external  InitialCondition=v0/0.3  SampleTime=-1  ICPrevOutput=DiscIntNeverNeededParam  ICPrevScaledInput=DiscIntNeverNeededParam
  Discrete-Time Integrator2 : DiscreteIntegrator  ExternalReset=sampled level  InitialConditionSource=external  InitialCondition=v0/0.3  SampleTime=-1  ICPrevOutput=DiscIntNeverNeededParam  ICPrevScaledInput=DiscIntNeverNeededParam
  Divide{,1,4..5} (4 alike) : Product  Inputs=*/
  Gain{,1..3} (4 alike) : Gain  Gain=0.5
  Product4 : Product  RndMeth=Zero
  Product5 : Product  RndMeth=Zero
  Unit Delay1 : UnitDelay  InitialCondition=par_VEH.r_stat0  SampleTime=-1
  Unit Delay2 : UnitDelay  InitialCondition=par_VEH.r_stat0  SampleTime=-1
  friction : Subsystem
  omega : Outport
  wires:
  friction/2(M_fric_R) -> Add1/4
  friction/1(M_fric_F) -> Add/4
  Bus Selector6/2 -> Unit Delay2/1  "<r_dyn_R>"
  Bus Selector6/1 -> Unit Delay1/1  "<r_dyn_F>"
  r_dyn/1 -> Bus Selector6/1
  Gain3/1 -> Add5/2  "M_brems_R"
  Gain1/1 -> Add5/1  "M_antr_R"
  Gain2/1 -> Add4/2  "M_brems_F"
  Gain/1 -> Add4/1  "M_antr_F"
  [Iwf] -> Divide/2
  Unit Delay2/1 -> Divide5/2
  Unit Delay1/1 -> Divide4/2
  Divide5/1 -> Discrete-Time Integrator1/3
  Divide4/1 -> Discrete-Time Integrator2/3
  Constant/1 -> Divide5/1, Divide4/1
  Divide1/1 -> Discrete-Time Integrator1/1  "omegap_R"
  Divide/1 -> Discrete-Time Integrator2/1  "omegap_F"
  Bus Selector3/2 -> Add1/1  "<Ms_R>"
  Bus Selector3/1 -> Add/1  "<Ms_F>"
  Fl/1 -> Bus Selector4/1
  My/1 -> Bus Selector3/1
  r_stat/1 -> Bus Selector2/1
  Add/1 -> Divide/1
  Add1/1 -> Divide1/1
  Add4/1 -> Add/2
  Add5/1 -> Add1/2
  Bus Selector4/1 -> Product4/1  "<Fl_F>"
  Bus Selector2/1 -> Product4/2  "<r_stat_F>"
  Bus Selector4/2 -> Product5/1  "<Fl_R>"
  Bus Selector2/2 -> Product5/2  "<r_stat_R>"
  Product4/1 -> Add/3
  Product5/1 -> Add1/3
  Bus Creator/1 -> friction/1(omega), omega/1
  Discrete-Time Integrator2/1 -> Bus Creator/1  "omega_F"
  Discrete-Time Integrator1/1 -> Bus Creator/2  "omega_R"
  [Iwr] -> Divide1/2
  [reset] -> Discrete-Time Integrator2/2, Discrete-Time Integrator1/2
  Bus Selector7/3 -> Add3/1  "<M_antr_RR>"
  Bus Selector8/3 -> Add7/1  "<M_brems_RR>"
  Bus Selector7/4 -> Add3/2  "<M_antr_LR>"
  Bus Selector8/4 -> Add7/2  "<M_brems_LR>"
  Bus Selector7/2 -> Add2/2  "<M_antr_LF>"
  Bus Selector8/1 -> Add6/1  "<M_brems_RF>"
  Bus Selector7/1 -> Add2/1  "<M_antr_RF>"
  M_brems/1 -> Bus Selector8/1
  M_antr/1 -> Bus Selector7/1
  Bus Selector8/2 -> Add6/2  "<M_brems_LF>"
  Add2/1 -> Gain/1
  Add3/1 -> Gain1/1
  Add6/1 -> Gain2/1
  Add7/1 -> Gain3/1

== system vehicle_model/simplified_vehicle_model/wheel/v0_korr ==
  vl : Inport
  r_dyn : Inport  Port=2
  omega : Inport  Port=3
  Bus Creator : BusCreator  Inputs=2
  Bus Selector1 : BusSelector  OutputSignals=r_dyn_F,r_dyn_R
  Bus Selector2 : BusSelector  OutputSignals=omega_F,omega_R
  Subsystem1 : Subsystem
  Subsystem2 : $bdroot/vehicle_model/wheel/v0_korr/Subsystem4  SystemSampleTime=-1
  v_low : Constant  Value=0.01  VectorParams1D=off
  omega_out : Outport
  wires:
  r_dyn/1 -> Bus Selector1/1
  omega/1 -> Bus Selector2/1
  Bus Creator/1 -> omega_out/1
  v_low/1 -> Subsystem1/2(v_low), Subsystem2/2
  Bus Selector1/1 -> Subsystem1/3(r_dyn)  "<r_dyn_F>"
  Bus Selector1/2 -> Subsystem2/3  "<r_dyn_R>"
  Bus Selector2/1 -> Subsystem1/4(omega)  "<omega_F>"
  Bus Selector2/2 -> Subsystem2/4  "<omega_R>"
  Subsystem1/1(omega_out) -> Bus Creator/1  "omega_F"
  Subsystem2/1 -> Bus Creator/2  "omega_R"
  vl/1 -> Subsystem2/1, Subsystem1/1(vl)
